simulink model "chap1_14"  (Simulink 6.3)
settings: Solver=ode45  StartTime=0.0  StopTime=1000  RelTol=1e-3
values from neighbouring files (symbols this model uses):
  kd = 0.01    [chap1_10.m]    (also in chap1_12.m = 10; chap1_13.m = 3; chap1_14int.m = 0.2; chap1_15.m = 0)
  ki = 2.0    (= 2)    [chap1_10.m]    (also in chap1_12.m = 0.1; chap1_13.m = 0.005; chap1_14int.m = 0.05; chap1_15.m = 9)
  kp = 1.0    (= 1)    [chap1_10.m]    (also in chap1_12.m = 8; chap1_13.m = 0.8; chap1_14int.m = 1.8; chap1_15.m = 0.85)
  ts = 0.001    [chap1_10.m]    (also in chap1_12.m; chap1_13.m = 20; chap1_14int.m = 20; chap1_15.m)
undefined symbols (not defined in the file or in its folder): den, DiscIntNeverNeededParam, num
settings Model: LastModifiedBy=Administrator  ExtModeTrigMode=oneshot  ExtModeArmWhenConnect=off  StrictBusMsg=None
settings DataIOCC: LimitDataPoints=off
settings OptimizationCC: BlockReduction=off  BooleanDataType=off
settings DebuggingCC: SolverPrmCheckMsg=none
settings HardwareCC: TargetUnknown=on

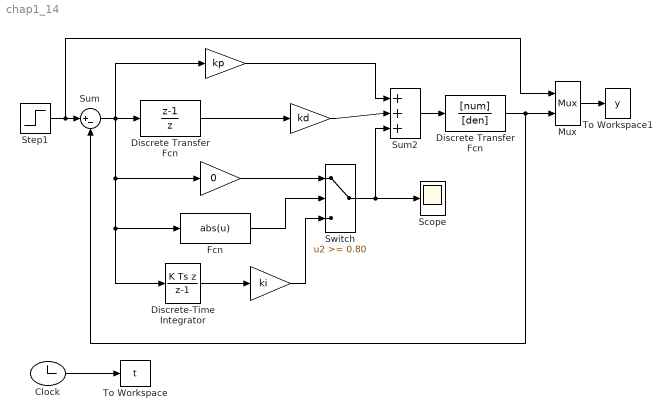
== system chap1_14 ==
  "  " : Gain  Gain=kp  SaturateOnIntegerOverflow=on
  "   " : Gain  Gain=ki  SaturateOnIntegerOverflow=on
  "    " : Gain  Gain=0  SaturateOnIntegerOverflow=on
  "     " : Gain  Gain=kd  SaturateOnIntegerOverflow=on
  Clock : Clock
      settings: Decimation=10
  Discrete Transfer Fcn : DiscreteTransferFcn  Numerator=[num]  Denominator=[den]  SampleTime=ts
  "Discrete Transfer Fcn " : DiscreteTransferFcn  Numerator=[1 -1]  Denominator=[1 0]  SampleTime=ts
  "Discrete-Time Integrator " : DiscreteIntegrator  IntegratorMethod=Integration: Backward Euler  SampleTime=ts  ICPrevOutput=DiscIntNeverNeededParam  ICPrevScaledInput=DiscIntNeverNeededParam
  Fcn : Fcn  Expr=abs(u)
  Mux : Mux  Inputs=2
  "Scope " : Scope
  Step1 : Step  Time=0  SampleTime=ts
  Sum : Sum  Inputs=|+-  SaturateOnIntegerOverflow=on  InputSameDT=on
  Sum2 : Sum  Inputs=|+++  SaturateOnIntegerOverflow=on  InputSameDT=on
  Switch : Switch  Threshold=0.80  SaturateOnIntegerOverflow=on  InputSameDT=on
  To Workspace : ToWorkspace  VariableName=t  SampleTime=-1  SaveFormat=Array
  To Workspace1 : ToWorkspace  VariableName=y  SampleTime=-1  SaveFormat=Array
  wires:
  "Discrete-Time Integrator "/1 -> "   "/1
  "    "/1 -> Switch/1
  Fcn/1 -> Switch/2
  "   "/1 -> Switch/3
  Mux/1 -> To Workspace1/1
  Discrete Transfer Fcn/1 -> Sum/2, Mux/2
  "  "/1 -> Sum2/1
  Sum2/1 -> Discrete Transfer Fcn/1
  Switch/1 -> "Scope "/1, Sum2/3
  "     "/1 -> Sum2/2
  "Discrete Transfer Fcn "/1 -> "     "/1
  Step1/1 -> Sum/1, Mux/1
  Sum/1 -> "  "/1, "    "/1, "Discrete-Time Integrator "/1, Fcn/1, "Discrete Transfer Fcn "/1
  Clock/1 -> To Workspace/1
